simulink model "Cascade"  (R2020a)
settings: Solver=ode14x  StartTime=0.0  StopTime=15  FixedStep=1e-3  RelTol=1e-3
values from neighbouring files (symbols this model uses):
  gain_P = ControlSystemDesignerSession.DesignerData.Designs.Data.C.K    [script_cascade.m]
  gain_V_I = gains_PI(2)    [script_cascade.m]
  gain_V_P = gains_PI(1)    [script_cascade.m]
settings Model: Creator=Admin  LastModifiedBy=Admin
settings DataIOCC: ReturnWorkspaceOutputsName=out_ffw

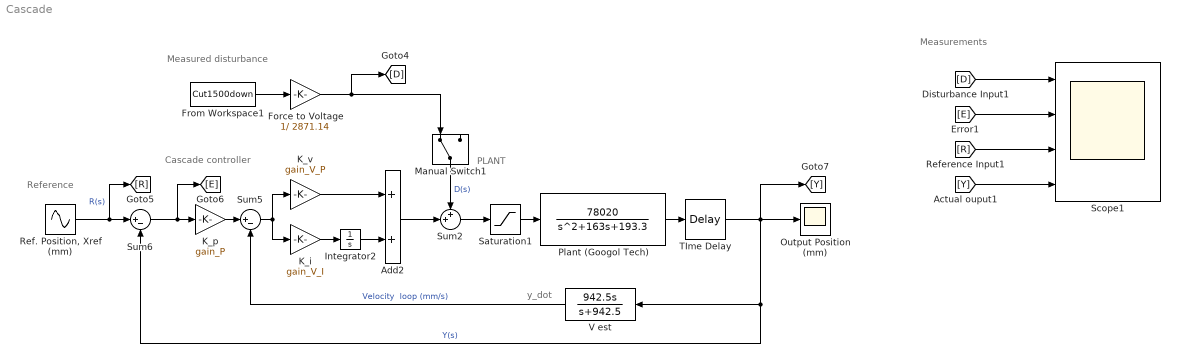
== system Cascade ==
  note: y_dot
  note: Reference
  note: Measured disturbance
  note: Measurements
  note: Cascade controller
  note: PLANT
  Add2 : Sum
  Force to Voltage : Gain  Gain=1/ 2871.14
  From Workspace1 : FromWorkspace  VariableName=Cut1500down  OutDataTypeStr=double  OutputAfterFinalValue=Setting to zero
  Integrator2 : Integrator  InitialCondition=.1
  K_i : Gain  Gain=gain_V_I
  K_p : Gain  Gain=gain_P
  K_v : Gain  Gain=gain_V_P
  Manual Switch1 : ManualSwitch
  Output Position (mm) : Scope
  Plant (Googol Tech) : TransferFcn  Numerator=[78020]  Denominator=[1 163 193.3]
  "Ref. Position, Xref (mm)" : Sin  Amplitude=5  Frequency=0.5*(2*pi)  SampleTime=0  Offset=1/2000
  Saturation1 : Saturate  UpperLimit=92  LowerLimit=-92
  Scope1 : Scope  NumInputPorts=4
  Sum2 : Sum  Inputs=++|
  Sum5 : Sum  Inputs=|+-
  Sum6 : Sum  Inputs=|+-
  TIme Delay : TransportDelay  DelayTime=0.0012
  V est : TransferFcn  Numerator=[942.5, 0]  Denominator=[1 942.5]
  wires:
  Force to Voltage/1 -> Manual Switch1/1, [D]
  Saturation1/1 -> Plant (Googol Tech)/1
  From Workspace1/1 -> Force to Voltage/1
  Manual Switch1/1 -> Sum2/1  "D(s)"
  [R] -> Scope1/3
  K_v/1 -> Add2/1
  Add2/1 -> Sum2/2
  [Y] -> Scope1/4
  [E] -> Scope1/2
  K_i/1 -> Integrator2/1
  [D] -> Scope1/1
  Sum5/1 -> K_v/1, K_i/1
  Sum2/1 -> Saturation1/1
  V est/1 -> Sum5/2  "Velocity  loop (mm/s)"
  "Ref. Position, Xref (mm)"/1 -> Sum6/1, [R]  "R(s)"
  Integrator2/1 -> Add2/2
  Sum6/1 -> K_p/1, [E]
  Plant (Googol Tech)/1 -> TIme Delay/1
  TIme Delay/1 -> Output Position (mm)/1, Sum6/2, V est/1, [Y]  "Y(s)"
  K_p/1 -> Sum5/1
